simulink model "pdl_linear_hw4n"  (R2017a)
settings: Solver=FixedStepAuto  StartTime=0.0  StopTime=duration  FixedStep=Ts  RelTol=1e-3
values from neighbouring files (symbols this model uses):
  A_a = [A E*Cw; zeros(2,4) Aw]    [pendulum_hw4linear.m]
  B_a = [B; zeros(2,1)]    [pendulum_hw4linear.m]
  C_a = [C zeros(2,2)]    [pendulum_hw4linear.m]
  E_a = [zeros(4,2); Bw]    [pendulum_hw4linear.m]
  f_p = 1e-4    (= 0.0001)    [pendulum_hw4linear.m]    (also in pendulum_hw4nonlinear.m)
  LC1_D = c2d(LC1_C,Ts)    [localcontroller.m]
  LC2_D = c2d(LC2_C,Ts)    [localcontroller.m]
  LC3_D = c2d(LC3_C,Ts)    [localcontroller.m]
  LC4_D = c2d(LC4_C,Ts)    [localcontroller.m]
  m_p = 1e-7    (= 1e-07)    [pendulum_hw4linear.m]    (also in pendulum_hw4nonlinear.m)
  Q_k = diag([5 2.5])    [pendulum_hw4linear.m]    (also in pendulum_hw4nonlinear.m = diag([1 1]))
  R_k = 1e-7*diag([1 1])    [pendulum_hw4linear.m]    (also in pendulum_hw4nonlinear.m = 1e-4*diag([1 1]))
  Ts = 0.001    [localcontroller.m]    (also in pendulum_hw4linear.m; pendulum_hw4nonlinear.m)
  w_p = 10    [pendulum_hw4linear.m]    (also in pendulum_hw4nonlinear.m)
  X_0 = [0;0*pi/180;0;0;0;0]    [pendulum_hw4linear.m]    (also in pendulum_hw4nonlinear.m = [0;0*pi/180;0;0])
undefined symbols (not defined in the file or in its folder): Delta, Gamma, Phi
libraries: simulink x3
settings Model: Creator=Salmon  LastModifiedBy=Salmon

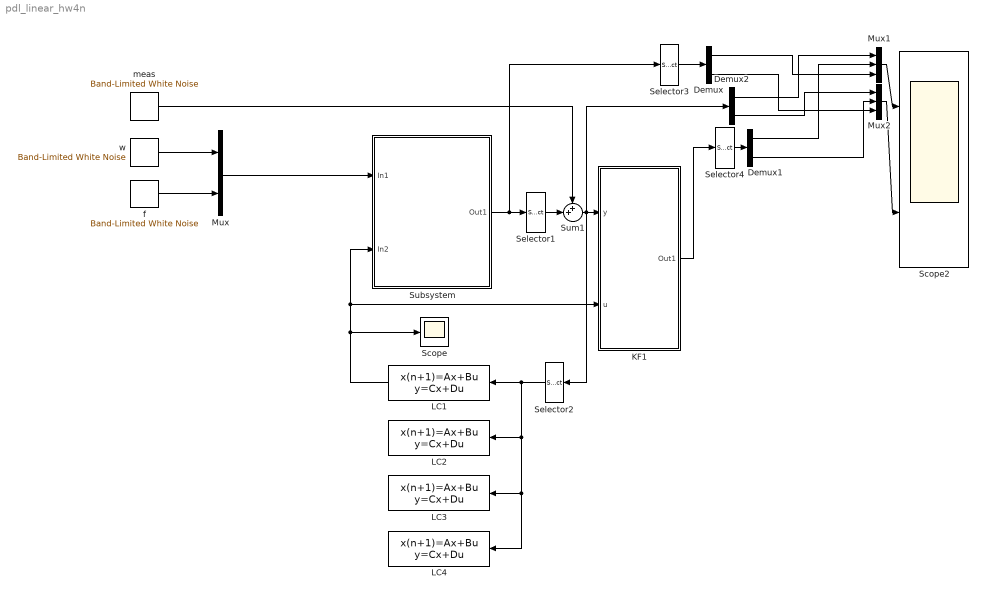
== system pdl_linear_hw4n ==
  Demux : Demux  Outputs=2
  Demux1 : Demux  Outputs=2
  Demux2 : Demux  Outputs=2
  KF1 : Subsystem
  LC1 : DiscreteStateSpace  A=LC1_D.A  B=LC1_D.B  C=LC1_D.C  D=LC1_D.D  SampleTime=Ts
  LC2 : DiscreteStateSpace  A=LC2_D.A  B=LC2_D.B  C=LC2_D.C  D=LC2_D.D  SampleTime=Ts
  LC3 : DiscreteStateSpace  A=LC3_D.A  B=LC3_D.B  C=LC3_D.C  D=LC3_D.D  SampleTime=Ts
  LC4 : DiscreteStateSpace  A=LC4_D.A  B=LC4_D.B  C=LC4_D.C  D=LC4_D.D  SampleTime=Ts
  Mux : Mux  Inputs=2
  Mux1 : Mux  Inputs=3
  Mux2 : Mux  Inputs=3
  Scope : Scope
  Scope2 : Scope  NumInputPorts=2
  Selector1 : Selector  InputPortWidth=6  IndexOptions=Index vector (dialog)  Indices=[1 2]  OutputSizes=1
  Selector2 : Selector  InputPortWidth=2  IndexOptions=Index vector (dialog)  Indices=[2 1]  OutputSizes=1
  Selector3 : Selector  InputPortWidth=6  IndexOptions=Index vector (dialog)  Indices=[1 2]  OutputSizes=1
  Selector4 : Selector  InputPortWidth=6  IndexOptions=Index vector (dialog)  Indices=[1 2]  OutputSizes=1
  Subsystem : Subsystem
  Sum1 : Sum  Inputs=++|
  f : simulink/Sources/Band-Limited White Noise  Cov=[f_p]  Ts=Ts  seed=[23341]
  meas : simulink/Sources/Band-Limited White Noise  Cov=[m_p,m_p]  Ts=Ts  seed=[123,23341]
  w : simulink/Sources/Band-Limited White Noise  Cov=[w_p]  Ts=Ts  seed=[23341]
  wires:
  w/1 -> Mux/1
  f/1 -> Mux/2
  Mux/1 -> Subsystem/1(In1)
  Subsystem/1(Out1) -> Selector1/1, Selector3/1
  LC1/1 -> Subsystem/2(In2), KF1/2(u), Scope/1
  Demux/1 -> Mux1/3
  Demux/2 -> Mux2/3
  Selector1/1 -> Sum1/2
  Demux1/1 -> Mux1/2
  KF1/1(Out1) -> Selector4/1
  Demux1/2 -> Mux2/2
  meas/1 -> Sum1/1
  Demux2/1 -> Mux1/1
  Demux2/2 -> Mux2/1
  Mux1/1 -> Scope2/1
  Mux2/1 -> Scope2/2
  Sum1/1 -> Selector2/1, Demux2/1, KF1/1(y)
  Selector2/1 -> LC3/1, LC4/1, LC2/1, LC1/1
  Selector3/1 -> Demux/1
  Selector4/1 -> Demux1/1

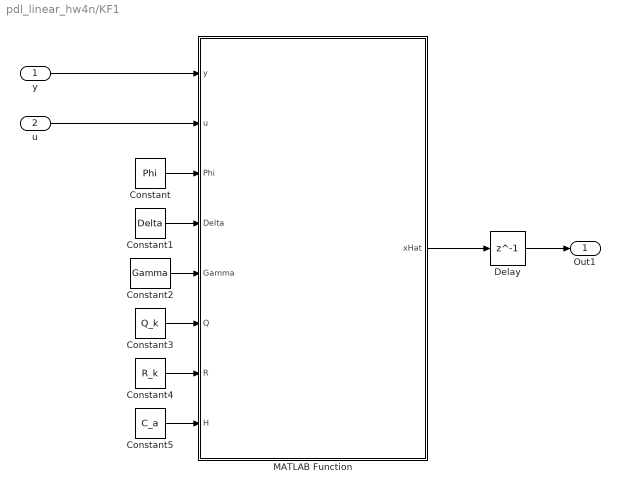
== system pdl_linear_hw4n/KF1 ==
  y : Inport
  u : Inport  Port=2
  Constant : Constant  Value=Phi
  Constant1 : Constant  Value=Delta
  Constant2 : Constant  Value=Gamma
  Constant3 : Constant  Value=Q_k
  Constant4 : Constant  Value=R_k
  Constant5 : Constant  Value=C_a
  Delay : Delay  DelayLength=1  InitialCondition=0
  MATLAB Function : MATLAB Function  TreatAsAtomicUnit=on
  Out1 : Outport
  wires:
  y/1 -> MATLAB Function/1(y)
  MATLAB Function/1(xHat) -> Delay/1
  u/1 -> MATLAB Function/2(u)
  Constant/1 -> MATLAB Function/3(Phi)
  Constant1/1 -> MATLAB Function/4(Delta)
  Constant3/1 -> MATLAB Function/6(Q)
  Constant2/1 -> MATLAB Function/5(Gamma)
  Constant4/1 -> MATLAB Function/7(R)
  Constant5/1 -> MATLAB Function/8(H)
  Delay/1 -> Out1/1

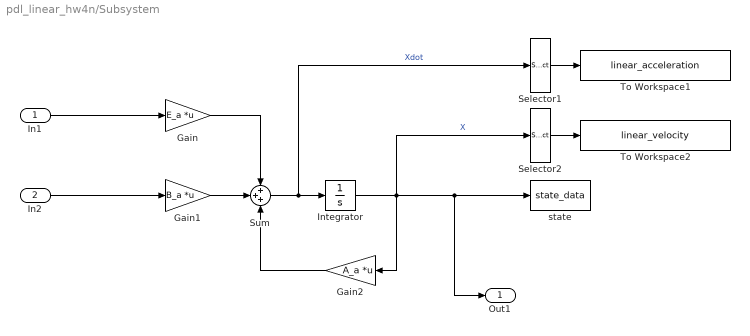
== system pdl_linear_hw4n/Subsystem ==
  In1 : Inport
  In2 : Inport  Port=2
  Gain : Gain  Gain=E_a  Multiplication=Matrix(K*u)
  Gain1 : Gain  Gain=B_a  Multiplication=Matrix(K*u)
  Gain2 : Gain  Gain=A_a  Multiplication=Matrix(K*u)
  Integrator : Integrator  InitialCondition=X_0
  Selector1 : Selector  InputPortWidth=6  IndexOptions=Index vector (dialog)  Indices=[3]  OutputSizes=1
  Selector2 : Selector  InputPortWidth=6  IndexOptions=Index vector (dialog)  Indices=[3]  OutputSizes=1
  Sum : Sum  Inputs=+++
  To Workspace1 : ToWorkspace  VariableName=linear_acceleration  SaveFormat=Structure With Time  SampleTime=-1
  To Workspace2 : ToWorkspace  VariableName=linear_velocity  SaveFormat=Structure With Time  SampleTime=-1
  state : ToWorkspace  VariableName=state_data  SaveFormat=Structure With Time  SampleTime=Ts
  Out1 : Outport
  wires:
  In1/1 -> Gain/1
  Gain/1 -> Sum/1
  Gain1/1 -> Sum/2
  Selector2/1 -> To Workspace2/1
  Selector1/1 -> To Workspace1/1
  Gain2/1 -> Sum/3
  In2/1 -> Gain1/1
  Integrator/1 -> Gain2/1, Selector2/1, Out1/1, state/1  "X"
  Sum/1 -> Integrator/1, Selector1/1  "Xdot"

== matlab function pdl_linear_hw4n/KF1/MATLAB Function ==
  data: y input; u input; xHat output; Phi input; Delta input; Gamma input; Q input; R input; H input
function xHat = fcn(y,u,Phi,Delta,Gamma,Q,R,H)

persistent Pbar xbar

% init. Pbar xbar
if isempty(Pbar)
    Pbar = 1e-6*eye(6);
end

if isempty(xbar)
    xbar = zeros(6,1);
end

% 1. Kalman gain
K = Pbar*H'*[H*Pbar*H'+R]^(-1);

% 2. state est. update
xHat = xbar + K*[y-H*xbar];

% 3. error covariance update
Phat = [eye(6)-K*H]*Pbar*[eye(6)-K*H]'+K*R*K';

% 4. state est. propagation
xbar = Phi*xHat+Delta*u;

% 5. error covariance propagation
Pbar = Phi*Phat*Phi'+Gamma*Q*Gamma';
